simulink model "PulsePickingModel"  (R2014a)
settings: Solver=FixedStepDiscrete  StartTime=0.0  StopTime=200.0  RelTol=1e-3
InitFcn:
  | initialization_pulsePicking;
StopFcn:
  | OutputPlotting;
libraries: BlockLib x3, dspsrcs4 x1
settings Model: Creator=Alexander  LastModifiedBy=Alexander

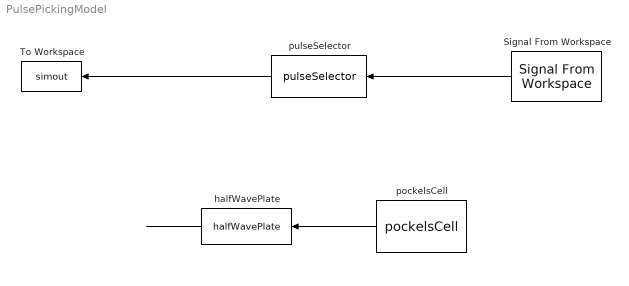
== system PulsePickingModel ==
  Signal From Workspace : dspsrcs4/Signal From Workspace  X=inputsignal  Ts=1  nsamps=1  OutputAfterFinalValue=Setting to zero  ignoreOrWarnInputAndFrameLengths=off
  To Workspace : ToWorkspace  VariableName=simout  SaveFormat=Timeseries  SampleTime=-1
  halfWavePlate : BlockLib/halfWavePlate  AxisAngle=pi/2
  pockelsCell : BlockLib/pockelsCell  OutputDimensions=1  AxisAngle=pi/4  PCID=PC1.ID
  pulseSelector : BlockLib/pulseSelector  OutputDimensions=1  PCID=PC1.ID
  wires:
  pockelsCell/1 -> halfWavePlate/1
  halfWavePlate/1 -> ?
  Signal From Workspace/1 -> pulseSelector/1
  pulseSelector/1 -> To Workspace/1
